simulink model "autosar_bsw_monitor"  (R2022b)
settings: Solver=FixedStepDiscrete  StartTime=0.0  StopTime=0.025  FixedStep=.005  MaxStep=.0001  RelTol=1e-3  EnableMultiTasking=on
undefined symbols (not defined in the file): Dem_EventStatusType
libraries: autosarlibdem x5
settings Model: Creator=The MathWorks, Inc.  LastModifiedBy=The MathWorks, Inc.
settings SolverCC: AlgebraicLoopSolver=TrustRegion  MaxZcPerStep=1
settings DataIOCC: LimitDataPoints=on  SaveFormat=Array  SignalLogging=off  DSMLogging=off  SaveTime=off  ReturnWorkspaceOutputs=off
settings OptimizationCC: DefaultParameterBehavior=Inlined  InlineInvariantSignals=on  EnhancedBackFolding=on  ExpressionDepthLimit=2147483647  StateBitsets=on  DataBitsets=on  ZeroExternalMemoryAtStartup=off  ZeroInternalMemoryAtStartup=off  NoFixptDivByZeroProtection=on  EfficientFloat2IntCast=on  EfficientMapNaN2IntZero=off  LifeSpan=1  BufferReusableBoundary=off  EfficientTunableParamExpr=on
settings DebuggingCC: SigSpecEnsureSampleTimeMsg=none  UnconnectedInputMsg=warning  UnconnectedOutputMsg=warning  UnconnectedLineMsg=warning  BusObjectLabelMismatch=none  AllowSymbolicDim=off  ModelReferenceSymbolNameMessage=none  StateNameClashWarn=warning  PregeneratedLibrarySubsystemCodeDiagnostic=none  StrictBusMsg=ErrorOnBusTreatedAsVector  SFUnexpectedBacktrackingDiag=warning  SFNoUnconditionalDefaultTransitionDiag=warning  SFExecutionAtInitializationDiag=none  SFMachineParentedDataDiag=warning  ArithmeticOperatorsInVariantConditions=warning
settings HardwareCC: TargetBitPerLong=64  TargetBitPerPointer=64  TargetBitPerSizeT=64  TargetBitPerPtrDiffT=64  TargetLongLongMode=on  TargetIntDivRoundTo=Zero  TargetEndianess=LittleEndian  TargetWordSize=64  TargetHWDeviceType=Generic->MATLAB Host Computer  ProdEqTarget=off
settings ModelReferenceCC: EnableRefExpFcnMdlSchedulingChecks=on  PropagateSignalLabelsOutOfModel=off
settings SFSimCC: SimUseLocalCustomCode=off  SimParseCustomCode=off  MATLABDynamicMemAlloc=off  CustomCodeUndefinedFunction=UseInterfaceOnly
settings RTWCC: Description=AUTOSAR  SystemTargetFile=autosar.tlc  GenCodeOnly=on  TemplateMakefile=ert_default_tmf  GenerateReport=on  RTWVerbose=off  RTWUseLocalCustomCode=off  IncludeHyperlinkInReport=on  LaunchReport=on  DLArmComputeVersion=19.05
settings CodeAppCC: ForceParamTrailComments=on  IgnoreCustomStorageClasses=off  IgnoreTestpoints=on  SimulinkDataObjDesc=on  CustomSymbolStrGlobalVar=rt$N$M  CustomSymbolStrType=$N$M  CustomSymbolStrFcn=$N$M$F  CustomSymbolStrMacro=$N$M  InsertBlockDesc=on  StateflowObjectComments=on  InternalIdentifier=Classic
settings STFCustomTargetCC: UtilityFuncGeneration=Shared location  ParMdlRefBuildCompliant=on  CompOptLevelCompliant=on  IncludeMdlTerminateFcn=off  CombineOutputUpdateFcns=on  SuppressErrorStatus=on  ERTCustomFileBanners=on  SupportNonFinite=off  SupportComplex=off  SupportContinuousTime=off  SupportNonInlinedSFcns=off  RemoveResetFunc=on  MATLABClassNameForMDSCustomization=Simulink.SoftwareTarget.ERTCustomization  CPPClassGenCompliant=on  AutosarCompliant=on  UseToolchainInfoCompliant=on  LookupTableObjectStructAxisOrder=2,1,3,4,...  LUTObjectStructOrderEvenSpacing=Size,Table,Breakpoints  SystemTargetFile=autosar.tlc
settings ERTTargetCC: UtilityFuncGeneration=Shared location  MultiwordLength=2048  ConcurrentExecutionCompliant=off  IncludeMdlTerminateFcn=off  SuppressErrorStatus=on  SupportNonFinite=off  SupportComplex=off  ModelStepFunctionPrototypeControlCompliant=off  AutosarCompliant=on  LookupTableObjectStructAxisOrder=2,1,3,4,...  LUTObjectStructOrderEvenSpacing=Size,Table,Breakpoints  ExtModeMexFile=noextcomm  InlinedParameterPlacement=NonHierarchical  ERTCustomFileTemplate=example_file_process.tlc  ERTFilePackagingFormat=CompactWithDataFile  ConvertIfToSwitch=off  SuppressUnreachableDefaultCases=off
settings ConfigComp: CovMetricSettings=dw  CovSaveCumulativeToWorkspaceVar=on  CovSaveSingleToWorkspaceVar=on  CovExternalEMLEnable=off

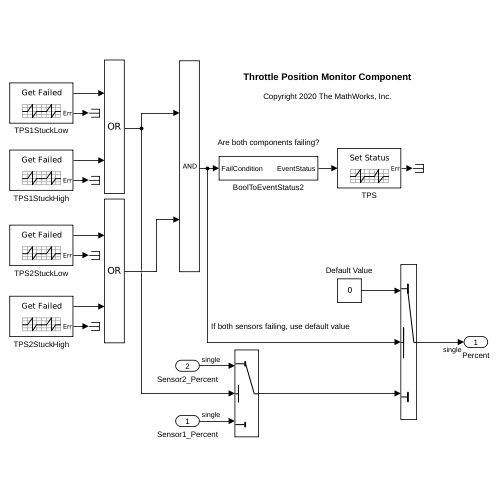
[thumbnail: Simulink's stored preview of the top-level diagram]
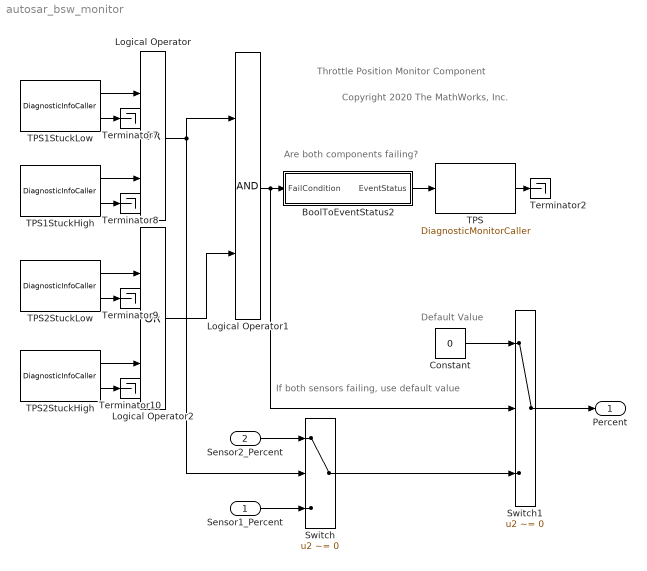
== system autosar_bsw_monitor ==
  note: Throttle Position Monitor Component
  note: Copyright 2020 The MathWorks, Inc.
  note: Default Value
  note: If both sensors failing, use default value
  note: Are both components failing?
  Sensor1_Percent : Inport  OutMin=0  OutMax=100  OutDataTypeStr=single  SampleTime=.005
  Sensor2_Percent : Inport  Port=2  OutMin=0  OutMax=100  OutDataTypeStr=single  SampleTime=.005
  BoolToEventStatus2 : Subsystem
  Constant : Constant  Value=0  OutDataTypeStr=single
  Logical Operator : Logic  Operator=OR  AllPortsSameDT=off  OutDataTypeStr=boolean
  Logical Operator1 : Logic  AllPortsSameDT=off  OutDataTypeStr=boolean
  Logical Operator2 : Logic  Operator=OR  AllPortsSameDT=off  OutDataTypeStr=boolean
  Switch : Switch  Criteria=u2 ~= 0  SaturateOnIntegerOverflow=off  InputSameDT=off
  Switch1 : Switch  Criteria=u2 ~= 0  SaturateOnIntegerOverflow=off  InputSameDT=off
  TPS : autosarlibdem/DiagnosticMonitorCaller  PortName=TPS  Operation=SetEventStatus  Datatype=Enum: Dem_EventStatusType  st=-1  ServiceImpl=autosar.bsw.DemDiagnosticMonitor
  TPS1StuckHigh : autosarlibdem/DiagnosticInfoCaller  PortName=TPS1StuckHigh  Operation=GetEventFailed  st=.005  ServiceImpl=autosar.bsw.DemDiagnosticInfo
  TPS1StuckLow : autosarlibdem/DiagnosticInfoCaller  PortName=TPS1StuckLow  Operation=GetEventFailed  st=.005  ServiceImpl=autosar.bsw.DemDiagnosticInfo
  TPS2StuckHigh : autosarlibdem/DiagnosticInfoCaller  PortName=TPS2StuckHigh  Operation=GetEventFailed  st=.005  ServiceImpl=autosar.bsw.DemDiagnosticInfo
  TPS2StuckLow : autosarlibdem/DiagnosticInfoCaller  PortName=TPS2StuckLow  Operation=GetEventFailed  st=.005  ServiceImpl=autosar.bsw.DemDiagnosticInfo
  Terminator{2,7..10} (5 alike) : Terminator
  Percent : Outport  OutMin=0  OutMax=100  OutDataTypeStr=single  SampleTime=.005  VectorParamsAs1DForOutWhenUnconnected=off
  wires:
  TPS2StuckHigh/2 -> Terminator10/1
  TPS1StuckLow/1 -> Logical Operator/1
  TPS2StuckLow/1 -> Logical Operator2/1
  TPS2StuckHigh/1 -> Logical Operator2/2
  TPS1StuckHigh/2 -> Terminator8/1
  BoolToEventStatus2/1(EventStatus) -> TPS/1
  Switch1/1 -> Percent/1
  Logical Operator1/1 -> Switch1/2, BoolToEventStatus2/1(FailCondition)
  TPS1StuckLow/2 -> Terminator7/1
  TPS1StuckHigh/1 -> Logical Operator/2
  Sensor2_Percent/1 -> Switch/1
  Constant/1 -> Switch1/1
  TPS/1 -> Terminator2/1
  Sensor1_Percent/1 -> Switch/3
  Logical Operator/1 -> Logical Operator1/1, Switch/2
  Switch/1 -> Switch1/3
  TPS2StuckLow/2 -> Terminator9/1
  Logical Operator2/1 -> Logical Operator1/2

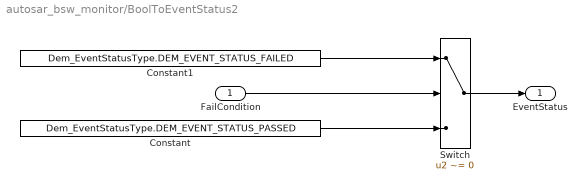
== system autosar_bsw_monitor/BoolToEventStatus2 ==
  FailCondition : Inport
  Constant : Constant  Value=Dem_EventStatusType.DEM_EVENT_STATUS_PASSED
  Constant1 : Constant  Value=Dem_EventStatusType.DEM_EVENT_STATUS_FAILED
  Switch : Switch  Criteria=u2 ~= 0  SaturateOnIntegerOverflow=off  InputSameDT=off
  EventStatus : Outport  VectorParamsAs1DForOutWhenUnconnected=off
  wires:
  Switch/1 -> EventStatus/1
  Constant1/1 -> Switch/1
  Constant/1 -> Switch/3
  FailCondition/1 -> Switch/2
